simulink model "rectgen_mod"  (R2018b)
settings: Solver=ode45  StartTime=0.0  StopTime=1.5  RelTol=1e-3  EnableMultiTasking=on
values from neighbouring files (symbols this model uses):
  a1 = R * C1    (= 0.05307)    [PT3_dat.m]
  a2 = L*(C1 + C2)    (= 0.000412)    [PT3_dat.m]
  a3 = R*L*C1*C2    (= 1.263066e-05)    [PT3_dat.m]
  s1 = 0.9    [PT3_dat.m]
  s2 = 0.1    [PT3_dat.m]
settings Model: Creator=wirth  LastModifiedBy=Peter
settings DataIOCC: LimitDataPoints=on  SaveFormat=Array  SignalLoggingSaveFormat=ModelDataLogs
settings OptimizationCC: ExpressionDepthLimit=2147483647  InitFltsAndDblsToZero=on  LifeSpan=inf
settings DebuggingCC: UnderspecifiedInitializationDetection=Classic  MergeDetectMultiDrivingBlocksExec=none  SolverPrmCheckMsg=warning  FcnCallInpInsideContextMsg=warning  StateNameClashWarn=warning  SFUnexpectedBacktrackingDiag=warning  SFNoUnconditionalDefaultTransitionDiag=warning  SFExecutionAtInitializationDiag=none
settings HardwareCC: ProdBitPerPointer=32  ProdBitPerSizeT=32  ProdBitPerPtrDiffT=32  ProdLargestAtomicFloat=None  ProdIntDivRoundTo=Undefined  ProdEndianess=Unspecified  ProdWordSize=32  ProdHWDeviceType=32-bit Generic
settings ModelReferenceCC: PropagateSignalLabelsOutOfModel=off
settings SFSimCC: SimUseLocalCustomCode=off
settings RTWCC: RTWUseLocalCustomCode=off
settings CodeAppCC: StateflowObjectComments=on
settings GRTTargetCC: TargetLangStandard=C89/C90 (ANSI)  GeneratePreprocessorConditionals=Disable all  CombineOutputUpdateFcns=off  GRTInterface=on
settings ConfigComp: CovMetricSettings=dw  CovHtmlReporting=on  CovSaveCumulativeToWorkspaceVar=on  CovSaveSingleToWorkspaceVar=on  CovExternalEMLEnable=off  CovSFcnEnable=off

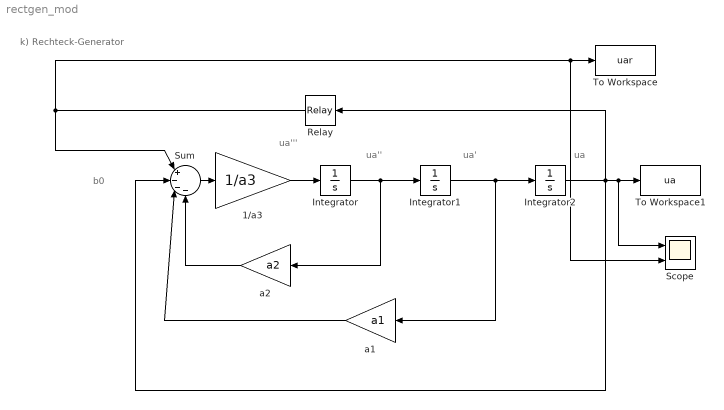
== system rectgen_mod ==
  note: ua'''
  note: ua
  note: ua''
  note: ua'
  note: k) Rechteck-Generator
  note: b0
  1/a3 : Gain  Gain=1/a3
  Integrator : Integrator
  Integrator1 : Integrator
  Integrator2 : Integrator
  Relay : Relay  OnSwitchValue=s1  OffSwitchValue=s2  OnOutputValue=ylow  OffOutputValue=yhigh
  Scope : Scope  NumInputPorts=2
  Sum : Sum  Inputs=|+---
  To Workspace : ToWorkspace  VariableName=uar  SampleTime=-1
  To Workspace1 : ToWorkspace  VariableName=ua  SampleTime=-1
  a1 : Gain  Gain=a1
  a2 : Gain  Gain=a2
  wires:
  Integrator2/1 -> Scope/1, To Workspace1/1, Relay/1, Sum/2
  Integrator/1 -> Integrator1/1, a2/1
  Integrator1/1 -> Integrator2/1, a1/1
  a1/1 -> Sum/3
  a2/1 -> Sum/4
  Relay/1 -> Scope/2, To Workspace/1, Sum/1
  1/a3/1 -> Integrator/1
  Sum/1 -> 1/a3/1
